simulink model "teensy_test"  (R2024a)
settings: Solver=ode4  StartTime=0.0  StopTime=10.0  FixedStep=0.0005  RelTol=1e-3
undefined symbols (not defined in the file or in its folder): CR, LF
libraries: instrumentseriallib x2, etargetslib x1
settings Model: Creator=gowon  LastModifiedBy=gowon

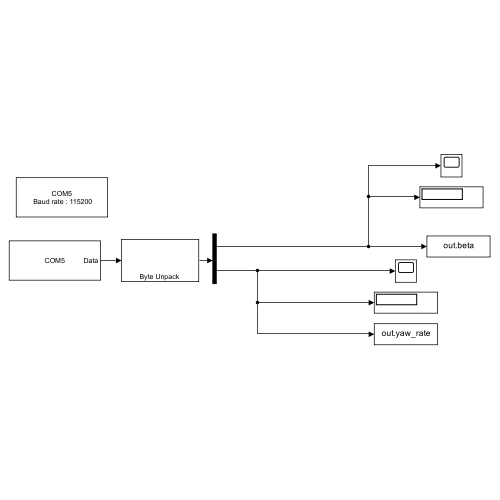
[thumbnail: Simulink's stored preview of the top-level diagram]
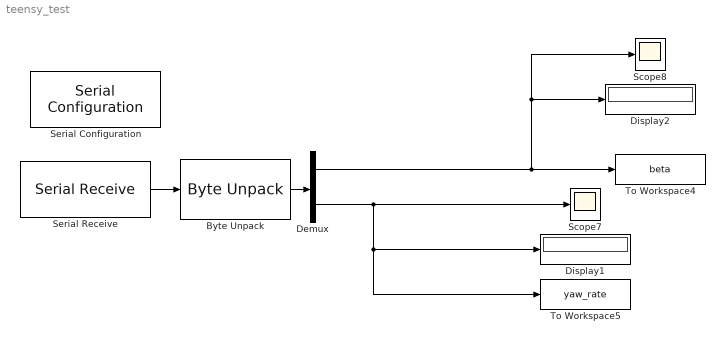
== system teensy_test ==
  Byte Unpack : etargetslib/Byte Unpack  dimensions={[2 1]}  datatypes={'single'}  byteAlign=4
      settings: LibrarySourceBlock=embeddedtargetslib/Host Communication/Byte Unpack
  Demux : Demux  Outputs=2
  Display1 : Display
  Display2 : Display
  Scope7 : Scope
  Scope8 : Scope
  Serial Configuration : instrumentseriallib/Serial Configuration  Priority=-200000  PortSel=COM5  Port=COM5  ComPort=COM5  BaudRate=115200  DataBits=8  Parity=none  StopBits=1  ByteOrder=little-endian  FlowControl=none  Timeout=10  SimulateUsing=Interpreted execution  BlockInModel=on  aMode=1
  Serial Receive : instrumentseriallib/Serial Receive  Priority=1  PortSel=COM5  Port=COM5  ComPort=COM5  DataType=uint8  SaveDataType=uint8  ToggleHeader=off  Header=[]  ToggleDataSize=on  DataSize=[1 8]  ToggleTerminator=off  Terminator=CR/LF ('\r\n')  CustomTerminator=[]  InputFormat=Column major  EnableBlockingMode=on  ActionDataUnavailable=Output last received value  ActionWhenDataUnavailable=Output last received value  CustomValue=0  SampleTime=0.0005  SimulateUsing=Interpreted execution  BlockInModel=on  aMode=1
  To Workspace4 : ToWorkspace  VariableName=beta  SaveFormat=Structure  SampleTime=-1
  To Workspace5 : ToWorkspace  VariableName=yaw_rate  SaveFormat=Structure  SampleTime=-1
  wires:
  Demux/2 -> Scope7/1, To Workspace5/1, Display1/1
  Byte Unpack/1 -> Demux/1
  Serial Receive/1 -> Byte Unpack/1
  Demux/1 -> Display2/1, Scope8/1, To Workspace4/1
